simulink model "simulink_discrete_2"  (Simulink 7.7)
settings: Solver=ode45  StartTime=0.0  StopTime=0.7  FixedStep=0.00001  MaxStep=0.00001  RelTol=1e-3
undefined symbols (not defined in the file or in its folder): T0, T1
libraries: cstblocks x6
settings Model: Creator=Koldo  LastModifiedBy=Koldo

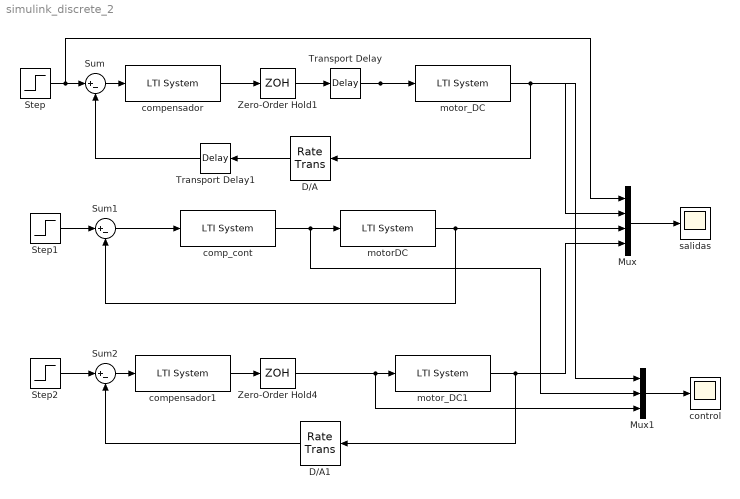
== system simulink_discrete_2 ==
  D/A : RateTransition  Integrity=off  Deterministic=off  X0=8.96  OutPortSampleTime=T1
  D/A1 : RateTransition  Integrity=off  Deterministic=off  X0=8.96  OutPortSampleTime=T1
  Mux : Mux
  Mux1 : Mux  Inputs=3
  Step : Step  Time=0.1  SampleTime=0
  Step1 : Step  Time=0.1  SampleTime=0
  Step2 : Step  Time=0.1  SampleTime=0
  Sum : Sum  Inputs=|+-
  Sum1 : Sum  Inputs=|+-
  Sum2 : Sum  Inputs=|+-
  Transport Delay : TransportDelay  DelayTime=T0/1.2
  Transport Delay1 : TransportDelay  DelayTime=0
  Zero-Order Hold1 : ZeroOrderHold  SampleTime=T1
  Zero-Order Hold4 : ZeroOrderHold  SampleTime=T1
  comp_cont : cstblocks/LTI System  SystemSampleTime=-1  sys=C  IC=[]
  compensador : cstblocks/LTI System  SystemSampleTime=-1  sys=CT0_tust  IC=[]
  compensador1 : cstblocks/LTI System  SystemSampleTime=-1  sys=CT0_tust  IC=[]
  control : Scope
      settings: MaxDataPoints=500000
  motorDC : cstblocks/LTI System  SystemSampleTime=-1  sys=G  IC=[]
  motor_DC : cstblocks/LTI System  SystemSampleTime=-1  sys=G  IC=[]
  motor_DC1 : cstblocks/LTI System  SystemSampleTime=-1  sys=G  IC=[]
  salidas : Scope
      settings: MaxDataPoints=500000
  wires:
  Step/1 -> Sum/1, Mux/1
  Sum/1 -> compensador/1
  motor_DC/1 -> Mux/2, D/A/1
  compensador/1 -> Zero-Order Hold1/1
  Step1/1 -> Sum1/1
  Sum1/1 -> comp_cont/1
  motorDC/1 -> Mux/3, Sum1/2
  comp_cont/1 -> motorDC/1, Mux1/2
  Mux/1 -> salidas/1
  Step2/1 -> Sum2/1
  Sum2/1 -> compensador1/1
  motor_DC1/1 -> Mux/4, D/A1/1
  Zero-Order Hold4/1 -> motor_DC1/1, Mux1/3
  Mux1/1 -> control/1
  D/A/1 -> Transport Delay1/1
  D/A1/1 -> Sum2/2
  compensador1/1 -> Zero-Order Hold4/1
  Zero-Order Hold1/1 -> Transport Delay/1
  Transport Delay/1 -> motor_DC/1, Mux1/1
  Transport Delay1/1 -> Sum/2
